simulink model "BehPlantLeanBroth"  (R2026a)
settings: Solver=VariableStepAuto  StopTime=14400
undefined symbols (not defined in the file): LB_PackRate_bph, LB_QCRate_bph, LB_Resupply_bph, LB_StaticPower_kW
settings Model: DataDictionary=BehParamsLeanBroth.sldd  Creator=sarah  LastModifiedBy=sarah

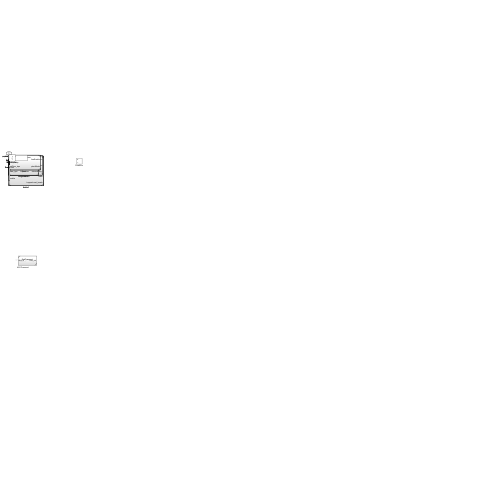
[thumbnail: Simulink's stored preview of the top-level diagram]
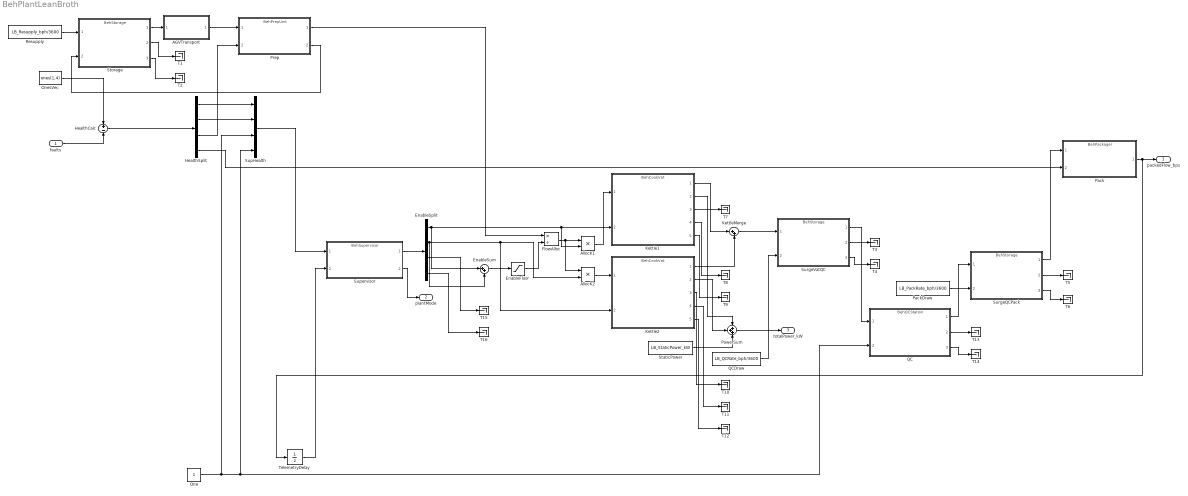
== system BehPlantLeanBroth ==
  faults : Inport  PortDimensions=4
  AGVTransport : Subsystem  ReferencedSubsystem=SubTransport
  AllocK1 : Product
  AllocK2 : Product
  EnableFloor : Saturate  UpperLimit=inf  LowerLimit=1
  EnableSplit : Demux
  EnableSum : Sum  Inputs=|++
  FlowAlloc : Product  Inputs=*/
  HealthCalc : Sum  Inputs=+-
  HealthSplit : Demux
  Kettle1 : ModelReference  ModelNameDialog=BehCookVat  UsingDefaultArgumentValue=0,0,0,0,0,0,0,0  SimulationMode=Normal  ModelReferenceVersion=1.4
  Kettle2 : ModelReference  ModelNameDialog=BehCookVat  UsingDefaultArgumentValue=0,0,0,0,0,0,0,0  SimulationMode=Normal  ModelReferenceVersion=1.4
  KettleMerge : Sum  Inputs=|++
  One : Constant
  OnesVec : Constant  Value=ones(1,4)
  Pack : ModelReference  ModelNameDialog=BehPackager  UsingDefaultArgumentValue=0,0  SimulationMode=Normal  ModelReferenceVersion=1.2
  PackDraw : Constant  Value=LB_PackRate_bph/3600
  PowerSum : Sum  Inputs=+++
  Prep : ModelReference  ModelNameDialog=BehPrepUnit  UsingDefaultArgumentValue=0,0  SimulationMode=Normal  ModelReferenceVersion=1.2
  QC : ModelReference  ModelNameDialog=BehQCStation  UsingDefaultArgumentValue=0,0,0,0  SimulationMode=Normal  ModelReferenceVersion=1.2
  QCDraw : Constant  Value=LB_QCRate_bph/3600
  Resupply : Constant  Value=LB_Resupply_bph/3600
  StaticPower : Constant  Value=LB_StaticPower_kW
  Storage : ModelReference  ModelNameDialog=BehStorage  UsingDefaultArgumentValue=0,0  SimulationMode=Normal  ModelReferenceVersion=1.2
  SupHealth : Mux
  Supervisor : ModelReference  ModelNameDialog=BehSupervisor  ParameterArgumentNames=NumLines  ParameterArgumentValues=LB_NumLines  UsingDefaultArgumentValue=0  SimulationMode=Normal  ModelReferenceVersion=1.3
  SurgeQCPack : ModelReference  ModelNameDialog=BehStorage  UsingDefaultArgumentValue=0,0  SimulationMode=Normal  ModelReferenceVersion=1.2
  SurgeVatQC : ModelReference  ModelNameDialog=BehStorage  UsingDefaultArgumentValue=0,0  SimulationMode=Normal  ModelReferenceVersion=1.2
  T{1..16} (16 alike) : Terminator
  TelemetryDelay : UnitDelay
  packedFlow_bps : Outport
  plantMode : Outport  Port=2
  totalPower_kW : Outport  Port=3
  wires:
  HealthCalc/1 -> HealthSplit/1
  Storage/3 -> T2/1
  Resupply/1 -> Storage/1
  SurgeQCPack/2 -> T5/1
  Kettle2/5 -> T12/1
  Kettle1/5 -> T9/1
  OnesVec/1 -> HealthCalc/1
  AGVTransport/1 -> Prep/1
  faults/1 -> HealthCalc/2
  Storage/2 -> T1/1
  QCDraw/1 -> SurgeVatQC/2
  Storage/1 -> AGVTransport/1
  Kettle2/2 -> PowerSum/2
  HealthSplit/1 -> SupHealth/1
  AllocK1/1 -> Kettle1/1
  HealthSplit/2 -> SupHealth/2
  Kettle2/4 -> T11/1
  HealthSplit/3 -> Prep/2
  HealthSplit/4 -> Pack/2
  One/1 -> SupHealth/4, QC/2, SupHealth/3
  TelemetryDelay/1 -> Supervisor/2
  Prep/1 -> FlowAlloc/1
  Supervisor/2 -> plantMode/1
  Prep/2 -> Storage/2
  SupHealth/1 -> Supervisor/1
  PackDraw/1 -> SurgeQCPack/2
  Supervisor/1 -> EnableSplit/1
  Kettle1/1 -> KettleMerge/1
  EnableSplit/1 -> AllocK1/2, Kettle1/2, EnableSum/1
  EnableSplit/2 -> AllocK2/2, Kettle2/2, EnableSum/2
  EnableSplit/3 -> T15/1
  QC/1 -> SurgeQCPack/1
  EnableSplit/4 -> T16/1
  EnableSum/1 -> EnableFloor/1
  SurgeVatQC/3 -> T4/1
  EnableFloor/1 -> FlowAlloc/2
  SurgeQCPack/3 -> T6/1
  FlowAlloc/1 -> AllocK2/1, AllocK1/1
  AllocK2/1 -> Kettle2/1
  Kettle1/2 -> PowerSum/1
  Kettle2/3 -> T10/1
  Kettle1/3 -> T7/1
  Kettle1/4 -> T8/1
  Kettle2/1 -> KettleMerge/2
  StaticPower/1 -> PowerSum/3
  KettleMerge/1 -> SurgeVatQC/1
  PowerSum/1 -> totalPower_kW/1
  SurgeVatQC/1 -> QC/1
  SurgeVatQC/2 -> T3/1
  QC/2 -> T13/1
  QC/3 -> T14/1
  SurgeQCPack/1 -> Pack/1
  Pack/1 -> TelemetryDelay/1, packedFlow_bps/1
